simulink model "CoVMD_TrqDesCoord"  (R2018a)
settings: configuration reference "cs_ert" (kept outside this file)
values from neighbouring files (symbols this model uses):
  VMD_swtVCMActv_C = 0    [CoVMD_TrqDesCoord.sldd]
undefined symbols (not defined in the file or in its folder): Switch
settings Model: DataDictionary=CoVMD_TrqDesCoord.sldd  Creator=zhoutinglin  LastModifiedBy=zhoutinglin

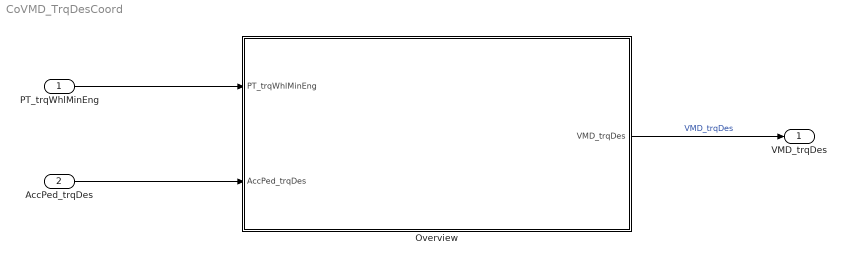
== system CoVMD_TrqDesCoord ==
  PT_trqWhlMinEng : Inport  Description=Minimum wheel torque from the engine  OutMin=-3000  OutMax=3000  OutDataTypeStr=Torq  Unit=Nm  PortDimensions=[1 1]
  AccPed_trqDes : Inport  Description=Driver torque value of propulsion after step limitation  Port=2  OutMin=-3000  OutMax=3000  OutDataTypeStr=Torq  Unit=Nm  PortDimensions=[1 1]
  Overview : Subsystem
  VMD_trqDes : Outport
  wires:
  PT_trqWhlMinEng/1 -> Overview/1(PT_trqWhlMinEng)
  AccPed_trqDes/1 -> Overview/2(AccPed_trqDes)
  Overview/1(VMD_trqDes) -> VMD_trqDes/1  "VMD_trqDes"

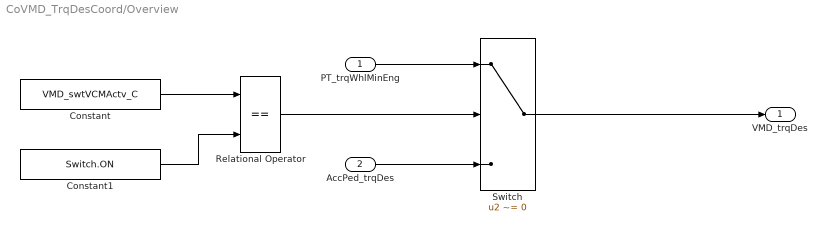
== system CoVMD_TrqDesCoord/Overview ==
  PT_trqWhlMinEng : Inport  Tag=Nm
  AccPed_trqDes : Inport  Tag=Nm  Port=2
  Constant : Constant  Value=VMD_swtVCMActv_C
  Constant1 : Constant  Value=Switch.ON
  Relational Operator : RelationalOperator  Operator===  OutDataTypeStr=boolean  RndMeth=Simplest
  Switch : Switch  Criteria=u2 ~= 0
  VMD_trqDes : Outport  Tag=Nm
  wires:
  Switch/1 -> VMD_trqDes/1
  AccPed_trqDes/1 -> Switch/3
  PT_trqWhlMinEng/1 -> Switch/1
  Relational Operator/1 -> Switch/2
  Constant1/1 -> Relational Operator/2
  Constant/1 -> Relational Operator/1
